simulink model "VCMGCM1962020b_v2"  (R2020b)
settings: Solver=FixedStepDiscrete  StartTime=0.0  StopTime=10.0  FixedStep=0.005  RelTol=1e-3  EnableMultiTasking=on
PreLoadFcn:
  | try, model_open; catch, disp('Error occurred while executing model pre-load callback: model_open.m'); disp('Please assure that the MATLAB working directory is set to the model directory before opening.'); end
InitFcn:
  | try, model_open; catch, end
undefined symbols (not defined in the file): Bridge, GCM, H, raptor_get_param_eval, raptor_get_safe_string, raptor_xcp_function
libraries: Blocks_lib x1165, Raptor_lib x665, simulink x62, VCM_lib x5
(part 4 of 23)

== system VCMGCM1962020b_v2/Fgnd/Control/Other/Cooling Pumps ==
  Data : Inport
  Bus Creator : BusCreator  Inputs=4
  Bus Selector1 : BusSelector  OutputSignals=Control.Mode.StartStop.ChgMode [Bool],Control.Mode.StartStop.RunMode [Bool]
  Bus Selector2 : BusSelector  OutputSignals=Control.Mode.StartStop.ChgMode [Bool],Control.Mode.StartStop.RunMode [Bool]
  Header : Blocks_lib/Header  width=Portrait  addtext=''
  Logical Operator : Logic  Inputs=3  AllPortsSameDT=off  OutDataTypeStr=boolean
  Logical Operator1 : Logic  Operator=OR  OutDataTypeStr=boolean
  Logical Operator2 : Logic  Inputs=3  AllPortsSameDT=off  OutDataTypeStr=boolean
  Logical Operator3 : Logic  Operator=OR  OutDataTypeStr=boolean
  Pump 1 Speed Request : Subsystem
  Pump 2 Speed Request : Subsystem
  raptor_adjustment : Raptor_lib/Data Storage/raptor_adjustment  paramName='CoolPump1EnblReqEnbl'  nameSource=Parameter  initValue=0  dataType=boolean  storage=Calibration  calDispType=Number  calEnum={'False', 'True'}  calGain=1  calOffset=0  calMax=inf  calMin=-inf  calFormat=''  calUnit='Bool'  calHelp='Cooling pump enable request enable'  calAccess=1  calFunction='Control | Cooling Loop'  calDispHeaders=off  calColHeaders={'Col1' 'Col2' 'Col3'}  calRowHeaders={'Row1' 'Row2' 'Row3'}
      settings: SourceProductName=Raptor
  raptor_adjustment1 : Raptor_lib/Data Storage/raptor_adjustment  paramName='CoolPump2EnblReqEnbl'  nameSource=Parameter  initValue=0  dataType=boolean  storage=Calibration  calDispType=Number  calEnum={'False', 'True'}  calGain=1  calOffset=0  calMax=inf  calMin=-inf  calFormat=''  calUnit='Bool'  calHelp='Cooling pump enable request enable'  calAccess=1  calFunction='Control | Cooling Loop'  calDispHeaders=off  calColHeaders={'Col1' 'Col2' 'Col3'}  calRowHeaders={'Row1' 'Row2' 'Row3'}
      settings: SourceProductName=Raptor
  Ctrl : Outport  VectorParamsAs1DForOutWhenUnconnected=off
  wires:
  Logical Operator1/1 -> Logical Operator/2
  Bus Selector1/1 -> Logical Operator1/1  "<ChgMode [Bool]>"
  Bus Selector1/2 -> Logical Operator1/2  "<RunMode [Bool]>"
  Bus Creator/1 -> Ctrl/1  "CoolPump"
  Pump 1 Speed Request/1(Bool) -> Logical Operator/3
  Logical Operator/1 -> Bus Creator/1  "CoolPump1EnblReq [Bool]"
  raptor_adjustment/1 -> Logical Operator/1
  Pump 1 Speed Request/2(%) -> Bus Creator/2  "CoolPump1SpdReq [%]"
  Pump 2 Speed Request/2(%) -> Bus Creator/4  "CoolPump2SpdReq [%]"
  raptor_adjustment1/1 -> Logical Operator2/1
  Pump 2 Speed Request/1(Bool) -> Logical Operator2/3
  Data/1 -> Bus Selector1/1, Pump 2 Speed Request/1(Data), Bus Selector2/1, Pump 1 Speed Request/1(Data)
  Bus Selector2/2 -> Logical Operator3/2  "<RunMode [Bool]>"
  Bus Selector2/1 -> Logical Operator3/1  "<ChgMode [Bool]>"
  Logical Operator3/1 -> Logical Operator2/2
  Logical Operator2/1 -> Bus Creator/3  "CoolPump2EnblReq [Bool]"

== system VCMGCM1962020b_v2/Fgnd/Control/Other/Heater ==
  Data : Inport
  Bus Creator : BusCreator  Inputs=3
  Bus Selector : BusSelector  OutputSignals=Control.Mode.StartStop.ChgMode [Bool],Control.Mode.StartStop.RunMode [Bool]
  Bus Selector1 : BusSelector  OutputSignals=VirtualSensors.Other.HeaterReq [Bool]
  Header : Blocks_lib/Header  width=Portrait  addtext=''
  Heater Pump : Stateflow chart  TreatAsAtomicUnit=on
  Logical Operator : Logic  Inputs=3  OutDataTypeStr=boolean
  Logical Operator1 : Logic  Operator=OR  OutDataTypeStr=boolean
  raptor_adjustment : Raptor_lib/Data Storage/raptor_adjustment  paramName='HeaterEnblReqEnbl'  nameSource=Parameter  initValue=0  dataType=boolean  storage=Calibration  calDispType=Number  calEnum={'False', 'True'}  calGain=1  calOffset=0  calMax=inf  calMin=-inf  calFormat=''  calUnit='Bool'  calHelp='Heater enable request enable'  calAccess=1  calFunction='Control | Heater'  calDispHeaders=off  calColHeaders={'Col1' 'Col2' 'Col3'}  calRowHeaders={'Row1' 'Row2' 'Row3'}
      settings: SourceProductName=Raptor
  raptor_adjustment1 : Raptor_lib/Data Storage/raptor_adjustment  paramName='HeaterOutletTempReq'  nameSource=Parameter  initValue=0  dataType=double  storage=Calibration  calDispType=Number  calEnum={'False', 'True'}  calGain=1.0  calOffset=0.0  calMax=inf  calMin=-inf  calFormat=''  calUnit='degC'  calHelp='Heater outlet temperature request'  calAccess=1  calFunction='Control | Heater'  calDispHeaders=off  calColHeaders={'Col1' 'Col2' 'Col3'}  calRowHeaders={'Row1' 'Row2' 'Row3'}
      settings: SourceProductName=Raptor
  raptor_adjustment2 : Raptor_lib/Data Storage/raptor_adjustment  paramName='HeaterPumpHoldTime'  nameSource=Parameter  initValue=0  dataType=uint16  storage=Calibration  calDispType=Number  calEnum={'Disabled', 'Enabled'}  calGain=samptime  calOffset=0  calMax=inf  calMin=-inf  calFormat='0.3'  calUnit='sec'  calHelp='Heater pump hold time (after heater turned off)'  calAccess=1  calFunction='Control | Heater'  calDispHeaders=off  calColHeaders={'Col1' 'Col2' 'Col3'}  calRowHeaders={'Row1' 'Row2' 'Row3'}
      settings: SourceProductName=Raptor
  raptor_adjustment3 : Raptor_lib/Data Storage/raptor_adjustment  paramName='HeaterPumpEnbl'  nameSource=Parameter  initValue=0  dataType=boolean  storage=Calibration  calDispType=Number  calEnum={'False', 'True'}  calGain=1  calOffset=0  calMax=inf  calMin=-inf  calFormat=''  calUnit='Bool'  calHelp='Heater pump enable'  calAccess=1  calFunction='Control | Heater'  calDispHeaders=off  calColHeaders={'Col1' 'Col2' 'Col3'}  calRowHeaders={'Row1' 'Row2' 'Row3'}
      settings: SourceProductName=Raptor
  Ctrl : Outport  VectorParamsAs1DForOutWhenUnconnected=off
  wires:
  Bus Selector1/1 -> Logical Operator/3  "<HeaterReq [Bool]>"
  Bus Creator/1 -> Ctrl/1  "Heater"
  Data/1 -> Bus Selector/1, Bus Selector1/1
  raptor_adjustment1/1 -> Bus Creator/2  "HeaterOutletTempReq [degC]"
  Bus Selector/2 -> Logical Operator1/2  "<RunMode [Bool]>"
  Bus Selector/1 -> Logical Operator1/1  "<ChgMode [Bool]>"
  Logical Operator1/1 -> Logical Operator/2
  raptor_adjustment/1 -> Logical Operator/1
  Heater Pump/1(Pump) -> Bus Creator/3  "HeaterPump [Bool]"
  raptor_adjustment2/1 -> Heater Pump/3(HoldTime)
  Logical Operator/1 -> Heater Pump/2(Heater), Bus Creator/1  "HeaterEnblReq [Bool]"
  raptor_adjustment3/1 -> Heater Pump/1(Enbl)

== system VCMGCM1962020b_v2/Fgnd/Control/Other/Other ==
  Data : Inport
  Bus Creator : BusCreator  Inputs=6
  Bus Selector : BusSelector  OutputSignals=Control.Mode.StartStop.OutptDiagEnbl [Bool]
  Bus Selector1 : BusSelector  OutputSignals=Control.Mode.StartStop.ModWake [Bool]
  Display : Subsystem
  FMWS : Subsystem
  Header : Blocks_lib/Header  width=Portrait  addtext=''
  Lights & Lamps : Subsystem
  Logical Operator : Logic  AllPortsSameDT=off  OutDataTypeStr=boolean
  Zero-Order Hold : ZeroOrderHold  SampleTime=-1
  raptor_adjustment : Raptor_lib/Data Storage/raptor_adjustment  paramName='HVILOutFrq_cal'  nameSource=Parameter  initValue=0  dataType=double  storage=Calibration  calDispType=Number  calEnum={'False', 'True'}  calGain=1.0  calOffset=0.0  calMax=inf  calMin=-inf  calFormat=''  calUnit='Hz'  calHelp='HVIL output frequency'  calAccess=1  calFunction='Control | Other'  calDispHeaders=off  calColHeaders={'Col1' 'Col2' 'Col3'}  calRowHeaders={'Row1' 'Row2' 'Row3'}
      settings: SourceProductName=Raptor
  raptor_adjustment1 : Raptor_lib/Data Storage/raptor_adjustment  paramName='SysWakeEnbl'  nameSource=Parameter  initValue=0  dataType=boolean  storage=Calibration  calDispType=Number  calEnum={'False', 'True'}  calGain=1  calOffset=0  calMax=inf  calMin=-inf  calFormat=''  calUnit='Bool'  calHelp='System wake enable'  calAccess=1  calFunction='Control | Other'  calDispHeaders=off  calColHeaders={'Col1' 'Col2' 'Col3'}  calRowHeaders={'Row1' 'Row2' 'Row3'}
      settings: SourceProductName=Raptor
  Ctrl : Outport  VectorParamsAs1DForOutWhenUnconnected=off
  wires:
  Bus Creator/1 -> Ctrl/1  "Other"
  Bus Selector/1 -> Zero-Order Hold/1  "<OutptDiagEnbl [Bool]>"
  Zero-Order Hold/1 -> Bus Creator/2  "MPDMWake [Bool]"
  raptor_adjustment/1 -> Bus Creator/1  "HVILOutFrq [Hz]"
  Lights & Lamps/1(Ctrl) -> Bus Creator/4
  Logical Operator/1 -> Bus Creator/3  "SysWake [Bool]"
  raptor_adjustment1/1 -> Logical Operator/1
  Data/1 -> Bus Selector1/1, FMWS/1(Data), Display/1(Data), Lights & Lamps/1(Data), Bus Selector/1
  Bus Selector1/1 -> Logical Operator/2  "<ModWake [Bool]>"
  Display/1(Ctrl) -> Bus Creator/5
  FMWS/1(Ctrl) -> Bus Creator/6

== system VCMGCM1962020b_v2/Fgnd/Control/Other/Park Pawl ==
  Data : Inport
  Bus Selector : BusSelector  OutputSignals=Control.Mode.PRNDMode [enum]
  CmprTo : Blocks_lib/CmprTo  op===  val='Prk'  enum=EnumLst.PRNDMode
  Header : Blocks_lib/Header  width=Portrait  addtext=''
  Logical Operator : Logic  OutDataTypeStr=boolean
  raptor_adjustment : Raptor_lib/Data Storage/raptor_adjustment  paramName='PrkPawlEnbl'  nameSource=Parameter  initValue=0  dataType=boolean  storage=Calibration  calDispType=Number  calEnum={'False', 'True'}  calGain=1  calOffset=0  calMax=inf  calMin=-inf  calFormat=''  calUnit='Bool'  calHelp='Park pawl enable'  calAccess=1  calFunction='Control | Park Pawl'  calDispHeaders=off  calColHeaders={'Col1' 'Col2' 'Col3'}  calRowHeaders={'Row1' 'Row2' 'Row3'}
      settings: SourceProductName=Raptor
  Bool : Outport  VectorParamsAs1DForOutWhenUnconnected=off
  wires:
  Data/1 -> Bus Selector/1
  Logical Operator/1 -> Bool/1
  Bus Selector/1 -> CmprTo/1  "<PRNDMode [enum]>"
  raptor_adjustment/1 -> Logical Operator/1
  CmprTo/1 -> Logical Operator/2

== system VCMGCM1962020b_v2/Fgnd/Control/Other/Power Steering Pump ==
  Data : Inport
  Bus Creator : BusCreator  Inputs=2
  Bus Selector : BusSelector  OutputSignals=Control.Mode.StartStop.RunMode [Bool],Control.Mode.PRNDMode [enum]
  Bus Selector1 : BusSelector  OutputSignals=VirtualSensors.Spd.VehSpd [kph]
  CmprTo : Blocks_lib/CmprTo  op=~=  val='Prk'  enum=EnumLst.PRNDMode
  Header : Blocks_lib/Header  width=Portrait  addtext=''
  Logical Operator : Logic  Inputs=3  OutDataTypeStr=boolean
  raptor_adjustment : Raptor_lib/Data Storage/raptor_adjustment  paramName='PSPInvtrEnblReqEnbl'  nameSource=Parameter  initValue=0  dataType=boolean  storage=Calibration  calDispType=Number  calEnum={'False', 'True'}  calGain=1  calOffset=0  calMax=inf  calMin=-inf  calFormat=''  calUnit='Bool'  calHelp='Power steering pump inverter enable request enable'  calAccess=1  calFunction='Control | Power Steering Pump'  calDispHeaders=off  calColHeaders={'Col1' 'Col2' 'Col3'}  calRowHeaders={'Row1' 'Row2' 'Row3'}
      settings: SourceProductName=Raptor
  raptor_table_1d : Raptor_lib/Table Lookup/raptor_table_1d  dataName='PSPMtrSpdReqTbl'  initValue=zeros(1,11)  dataType=double  storage=Calibration  initValueX=[1:11]  dataTypeXY=double  storageXY=Calibration  calVisible=on  showTable=on  calGain=1.0  calOffset=0.0  calMax=Inf  calMin=-Inf  calFormat='-1'  calUnit='rpm'  calHelp='Power steering pump motor speed request'  showBreakpoint=on  dataNameX='VehSpd11IdxArr'  calGainX=1.0  calOffsetX=0.0  calMaxX=Inf  calMinX=-Inf  calFormatX='-1'  calUnitX='kph'  calHelpX='Index array'  calAccess=1  calFunction='Control | Power Steering Pump'  measureEnable=on  mName='PSPMtrSpdReq'
      settings: SourceProductName=Raptor
  Ctrl : Outport  VectorParamsAs1DForOutWhenUnconnected=off
  wires:
  CmprTo/1 -> Logical Operator/3
  raptor_table_1d/1 -> Bus Creator/2  "PSPMtrSpdReq [rpm]"
  Logical Operator/1 -> Bus Creator/1  "PSPInvtrEnblReq [Bool]"
  Bus Creator/1 -> Ctrl/1  "PSPInvtr"
  Bus Selector1/1 -> raptor_table_1d/1  "<VehSpd [kph]>"
  Data/1 -> Bus Selector/1, Bus Selector1/1
  Bus Selector/1 -> Logical Operator/2  "<RunMode [Bool]>"
  Bus Selector/2 -> CmprTo/1  "<PRNDMode [enum]>"
  raptor_adjustment/1 -> Logical Operator/1

== system VCMGCM1962020b_v2/Fgnd/Control/PDU/High-Voltage Discharge Contactor ==
  Data : Inport
  Bus Selector : BusSelector  OutputSignals=Control.Mode.StartStop.HVDschg [Bool]
  HV Discharge : Stateflow chart  TreatAsAtomicUnit=on
  Header : Blocks_lib/Header  width=Portrait  addtext=''
  raptor_adjustment1 : Raptor_lib/Data Storage/raptor_adjustment  paramName='HVDschgMxTime'  nameSource=Parameter  initValue=0  dataType=uint16  storage=Calibration  calDispType=Number  calEnum={'Disabled', 'Enabled'}  calGain=samptime  calOffset=0  calMax=inf  calMin=-inf  calFormat='0.3'  calUnit='sec'  calHelp='High-voltage discharge maximum time (before setting fault)'  calAccess=1  calFunction='Control | PDU'  calDispHeaders=off  calColHeaders={'Col1' 'Col2' 'Col3'}  calRowHeaders={'Row1' 'Row2' 'Row3'}
      settings: SourceProductName=Raptor
  raptor_adjustment2 : Raptor_lib/Data Storage/raptor_adjustment  paramName='HVDschgRetryWaitTime'  nameSource=Parameter  initValue=0  dataType=uint16  storage=Calibration  calDispType=Number  calEnum={'Disabled', 'Enabled'}  calGain=samptime  calOffset=0  calMax=inf  calMin=-inf  calFormat='0.3'  calUnit='sec'  calHelp='High-voltage discharge retry wait time (after fault)'  calAccess=1  calFunction='Control | PDU'  calDispHeaders=off  calColHeaders={'Col1' 'Col2' 'Col3'}  calRowHeaders={'Row1' 'Row2' 'Row3'}
      settings: SourceProductName=Raptor
  Bool : Outport  VectorParamsAs1DForOutWhenUnconnected=off
  wires:
  Data/1 -> Bus Selector/1
  raptor_adjustment1/1 -> HV Discharge/2(MxTime)
  raptor_adjustment2/1 -> HV Discharge/3(RetryWaitTime)
  Bus Selector/1 -> HV Discharge/1(Enbl)  "<HVDschg [Bool]>"
  HV Discharge/1(Cntr) -> Bool/1

== system VCMGCM1962020b_v2/Fgnd/Control/PDU/Main  Contactor Cmd ==
  Data : Inport
  BusCreator : BusCreator  Inputs=2
  Enable : Subsystem
  HV Detect : Subsystem
  Header : Blocks_lib/Header  width=Portrait  addtext=''
  PreCharge Sequence : Stateflow chart  TreatAsAtomicUnit=on
  raptor_adjustment1 : Raptor_lib/Data Storage/raptor_adjustment  paramName=[nam 'PreChgMxTime']  nameSource=Parameter  initValue=0  dataType=uint16  storage=Calibration  calDispType=Number  calEnum={'Disabled', 'Enabled'}  calGain=samptime  calOffset=0  calMax=inf  calMin=-inf  calFormat='0.3'  calUnit='sec'  calHelp='Pre-charge maximum time (before setting fault)'  calAccess=1  calFunction=group  calDispHeaders=off  calColHeaders={'Col1' 'Col2' 'Col3'}  calRowHeaders={'Row1' 'Row2' 'Row3'}
      settings: SourceProductName=Raptor
  raptor_adjustment2 : Raptor_lib/Data Storage/raptor_adjustment  paramName=[nam 'PreChgRetryWaitTime']  nameSource=Parameter  initValue=0  dataType=uint16  storage=Calibration  calDispType=Number  calEnum={'Disabled', 'Enabled'}  calGain=samptime  calOffset=0  calMax=inf  calMin=-inf  calFormat='0.3'  calUnit='sec'  calHelp='Pre-charge retry wait time (after fault)'  calAccess=1  calFunction=group  calDispHeaders=off  calColHeaders={'Col1' 'Col2' 'Col3'}  calRowHeaders={'Row1' 'Row2' 'Row3'}
      settings: SourceProductName=Raptor
  raptor_adjustment3 : Raptor_lib/Data Storage/raptor_adjustment  paramName=[nam 'PreChgMxAttempts']  nameSource=Parameter  initValue=0  dataType=uint16  storage=Calibration  calDispType=Number  calEnum={'Disabled', 'Enabled'}  calGain=1  calOffset=0  calMax=inf  calMin=-inf  calFormat=''  calUnit='count'  calHelp='Pre-charge maximum attempts'  calAccess=1  calFunction=group  calDispHeaders=off  calColHeaders={'Col1' 'Col2' 'Col3'}  calRowHeaders={'Row1' 'Row2' 'Row3'}
      settings: SourceProductName=Raptor
  raptor_measurement : Raptor_lib/Data Storage/raptor_measurement  paramName=[nam 'MainCntrClosed']  nameSource=Parameter  calDispType=Number  calEnum={}  calGain=1.0  calOffset=0.0  calMax=inf  calMin=-inf  calFormat='-1'  calUnit='Bool'  calHelp='Main Cntr complete'  calAccess=1  calFunction=group  calVisible=on
      settings: SourceProductName=Raptor
  Ctrl : Outport  VectorParamsAs1DForOutWhenUnconnected=off
  wires:
  Data/1 -> Enable/1(Data), HV Detect/1(Data)
  raptor_adjustment3/1 -> PreCharge Sequence/5(MxAttempts)
  raptor_adjustment2/1 -> PreCharge Sequence/4(RetryWaitTime)
  raptor_adjustment1/1 -> PreCharge Sequence/3(MxTime)
  PreCharge Sequence/1(Complete) -> BusCreator/1, raptor_measurement/1  "MainPreChgComplete [Bool]"
  Enable/1(Bool) -> PreCharge Sequence/1(Enbl)  "MainPosCntr [Bool]"
  BusCreator/1 -> Ctrl/1  "MainCntrs"
  HV Detect/1(Full) -> PreCharge Sequence/2(HVDetect)
  PreCharge Sequence/2(CntrCmd) -> BusCreator/2  "MainPreChgCntr [Bool]"

== system VCMGCM1962020b_v2/Fgnd/Control/PDU/PDU Contactor Commands ==
  note: This Logic Determins if Contactors are commanded and confirmed
  Data : Inport
  BusCreator : BusCreator  Inputs=7
  CntrStatus : Subsystem
  Drive Inverter Contactor : Subsystem
  Enable : Subsystem
  HV Detect : Subsystem
  Header : Blocks_lib/Header  width=Portrait  addtext=''
  OR : Logic  Operator=OR  AllPortsSameDT=off  OutDataTypeStr=boolean
  Zero-Order Hold1 : ZeroOrderHold  SampleTime=-1
  Zero-Order Hold2 : ZeroOrderHold  SampleTime=-1
  Ctrl : Outport  VectorParamsAs1DForOutWhenUnconnected=off
  wires:
  Data/1 -> Drive Inverter Contactor/1(Data), Enable/1(Data), CntrStatus/1(Data), HV Detect/1(Data)
  Enable/1(RunEnbl) -> BusCreator/2, OR/1  "RunCntrs [Bool]"
  BusCreator/1 -> Ctrl/1  "PDUCntrs"
  Enable/2(ChrgEnbl) -> Zero-Order Hold2/1, OR/2  "ChrgCntr"
  Drive Inverter Contactor/1(Bool) -> BusCreator/1  "DrvInvtrCntrCmd [Bool]"
  Zero-Order Hold1/1 -> BusCreator/3  "DCDCCntrCmd [Bool]"
  OR/1 -> Zero-Order Hold1/1
  Zero-Order Hold2/1 -> BusCreator/4  "ChrgrCntrCmd [Bool]"
  HV Detect/1(Full) -> BusCreator/5  "HVDetected[Bool}"
  CntrStatus/1(RunClosed) -> BusCreator/6  "RunCntrsClosed [Bool]"
  CntrStatus/2(ChrgClosed) -> BusCreator/7  "ChrgCntrsClosed [Bool]"

== system VCMGCM1962020b_v2/Fgnd/Diagnostics/Diagnostics/A//C Compressor Fault ==
  Data : Inport
  Bus Selector : BusSelector  OutputSignals=Sensors.CAN.Other.ACC.ACCSTATUS1.ACCFltStat.ACCFltStatVld [Bool],VirtualSensors.PDU.MainCntrClosedVld [Bool]
  EvalDiag : Subsystem
  Header : Blocks_lib/Header  width=Portrait  addtext=''
  Logical Operator : Logic  AllPortsSameDT=off  OutDataTypeStr=boolean
  wires:
  Data/1 -> EvalDiag/1(Data), Bus Selector/1
  Bus Selector/1 -> Logical Operator/1  "<ACCFltStatVld [Bool]>"
  Bus Selector/2 -> Logical Operator/2  "<MainCntrClosedVld [Bool]>"
  Logical Operator/1 -> EvalDiag/Enable

== system VCMGCM1962020b_v2/Fgnd/Diagnostics/Diagnostics/Battery Cell Temperature (avg) High  ==
  Data : Inport
  Bus Selector : BusSelector  OutputSignals=VirtualSensors.Batt.BattCellTempAvgVld [Bool]
  EvalDiag : Subsystem
  Header : Blocks_lib/Header  width=Portrait  addtext=''
  wires:
  Bus Selector/1 -> EvalDiag/Enable  "<BattCellTempAvgVld [Bool]>"
  Data/1 -> Bus Selector/1, EvalDiag/1(Data)

== system VCMGCM1962020b_v2/Fgnd/Diagnostics/Diagnostics/Battery Cell Temperature (max) High ==
  Data : Inport
  Bus Selector : BusSelector  OutputSignals=VirtualSensors.Batt.BattCellTempMxVld [Bool]
  EvalDiag : Subsystem
  Header : Blocks_lib/Header  width=Portrait  addtext=''
  wires:
  Data/1 -> EvalDiag/1(Data), Bus Selector/1
  Bus Selector/1 -> EvalDiag/Enable  "<BattCellTempMxVld [Bool]>"

== system VCMGCM1962020b_v2/Fgnd/Diagnostics/Diagnostics/Battery Cell Voltage (max) High ==
  Data : Inport
  Bus Selector : BusSelector  OutputSignals=VirtualSensors.Batt.BattCellVoltMxVld [Bool]
  EvalDiag : Subsystem
  Header : Blocks_lib/Header  width=Portrait  addtext=''
  wires:
  Bus Selector/1 -> EvalDiag/Enable  "<BattCellVoltMxVld [Bool]>"
  Data/1 -> Bus Selector/1, EvalDiag/1(Data)

== system VCMGCM1962020b_v2/Fgnd/Diagnostics/Diagnostics/Battery Cell Voltage (min) Low ==
  Data : Inport
  Bus Selector : BusSelector  OutputSignals=VirtualSensors.Batt.BattCellVoltMnVld [Bool]
  EvalDiag : Subsystem
  Header : Blocks_lib/Header  width=Portrait  addtext=''
  wires:
  Data/1 -> EvalDiag/1(Data), Bus Selector/1
  Bus Selector/1 -> EvalDiag/Enable  "<BattCellVoltMnVld [Bool]>"

== system VCMGCM1962020b_v2/Fgnd/Diagnostics/Diagnostics/Battery Current High ==
  Data : Inport
  Bus Selector : BusSelector  OutputSignals=VirtualSensors.Batt.BattCurVld [Bool],VirtualSensors.Batt.BattDCLVld [Bool],VirtualSensors.Batt.BattCCLVld [Bool]
  EvalDiag : Subsystem
  Header : Blocks_lib/Header  width=Portrait  addtext=''
  Logical Operator : Logic  Inputs=3  AllPortsSameDT=off  OutDataTypeStr=boolean
  wires:
  Data/1 -> EvalDiag/1(Data), Bus Selector/1
  Bus Selector/3 -> Logical Operator/3  "<BattCCLVld [Bool]>"
  Bus Selector/1 -> Logical Operator/1  "<BattCurVld [Bool]>"
  Bus Selector/2 -> Logical Operator/2  "<BattDCLVld [Bool]>"
  Logical Operator/1 -> EvalDiag/Enable

== system VCMGCM1962020b_v2/Fgnd/Diagnostics/Diagnostics/Battery Fault ==
  Data : Inport
  Bus Selector : BusSelector  OutputSignals=VirtualSensors.Batt.BattFaultVld [Bool]
  EvalDiag : Subsystem
  Header : Blocks_lib/Header  width=Portrait  addtext=''
  wires:
  Data/1 -> Bus Selector/1, EvalDiag/1(Data)
  Bus Selector/1 -> EvalDiag/Enable  "<BattFaultVld [Bool]>"

== system VCMGCM1962020b_v2/Fgnd/Diagnostics/Diagnostics/CAN Bus Passive ==
  Data : Inport
  Bus Selector : BusSelector  OutputSignals=Control.Mode.StartStop.CANDiagEnbl [Bool]
  EvalDiag : Subsystem
  Header : Blocks_lib/Header  width=Portrait  addtext=''
  wires:
  Data/1 -> Bus Selector/1
  Bus Selector/1 -> EvalDiag/Enable  "<CANDiagEnbl [Bool]>"

== system VCMGCM1962020b_v2/Fgnd/Diagnostics/Diagnostics/Charger (off-board) Isolation Fault ==
  Data : Inport
  Bus Selector : BusSelector  OutputSignals=VirtualSensors.Chgr.OffBoard.OffBoardChgrIsoFaultVld [Bool]
  EvalDiag : Subsystem
  Header : Blocks_lib/Header  width=Portrait  addtext=''
  wires:
  Data/1 -> Bus Selector/1, EvalDiag/1(Data)
  Bus Selector/1 -> EvalDiag/Enable  "<OffBoardChgrIsoFaultVld [Bool]>"

== system VCMGCM1962020b_v2/Fgnd/Diagnostics/Diagnostics/Charger (on-board) Fault ==
  Data : Inport
  Bus Selector : BusSelector  OutputSignals=VirtualSensors.Chgr.OnBoard.OnBoardChgrFaultVld [Bool]
  EvalDiag : Subsystem
  Header : Blocks_lib/Header  width=Portrait  addtext=''
  wires:
  Data/1 -> Bus Selector/1, EvalDiag/1(Data)
  Bus Selector/1 -> EvalDiag/Enable  "<OnBoardChgrFaultVld [Bool]>"

== system VCMGCM1962020b_v2/Fgnd/Diagnostics/Diagnostics/Contactor SOH Faults ==
  Data : Inport
  Bus Selector : BusSelector  OutputSignals=VirtualSensors.PDU.MainPosCntrClosedVld [Bool],VirtualSensors.Batt.BattCurVld [Bool],VirtualSensors.PDU.MainPosCntrClosed [Bool],VirtualSensors.Batt.BattCur [A]
  Bus Selector1 : BusSelector  Commented=on  OutputSignals=VirtualSensors.PDU.MainNegCntrClosedVld [Bool],VirtualSensors.Batt.BattCurVld [Bool],VirtualSensors.PDU.MainNegCntrClosed [Bool],VirtualSensors.Batt.BattCur [A]
  Bus Selector2 : BusSelector  OutputSignals="VirtualSensors.PDU.DCDCCntrClosedVld  [Bool],VirtualSensors.Chgr.OffBoard.OffBoardChgrDCCurVld [Bool],VirtualSensors.PDU.DCDCCntrClosed [Bool],VirtualSensors.Chgr.OffBoard.OffBoardChgrDCCur [A]"
  Bus Selector3 : BusSelector  Commented=on  OutputSignals=VirtualSensors.PDU.DCChgNegCntrClosedVld [Bool],VirtualSensors.Chgr.OffBoard.OffBoardChgrDCCurVld [Bool],VirtualSensors.PDU.DCChgNegCntrClosed [Bool],VirtualSensors.Chgr.OffBoard.OffBoardChgrDCCur [A]
  Bus Selector4 : BusSelector  Commented=on  OutputSignals=VirtualSensors.PDU.DrvInvtrCntrClosedVld [Bool],VirtualSensors.DrvInvtr.DrvInvtrCurVld [Bool],VirtualSensors.PDU.DrvInvtrCntrClosed [Bool],VirtualSensors.DrvInvtr.DrvInvtrCur [A]
  CntrFltSOH : VCM_lib/CntrFltSOH  nam='MainPosCntr'  len=9  group='Diagnostics | System'  samptime=samptime
  CntrFltSOH1 : VCM_lib/CntrFltSOH  Commented=on  nam='MainNegCntr'  len=9  group='Diagnostics | System'  samptime=samptime
  CntrFltSOH2 : VCM_lib/CntrFltSOH  nam='DCChgPosCntr'  len=9  group='Diagnostics | System'  samptime=samptime
  CntrFltSOH3 : VCM_lib/CntrFltSOH  Commented=on  nam='DCChgNegCntr'  len=9  group='Diagnostics | System'  samptime=samptime
  CntrFltSOH4 : VCM_lib/CntrFltSOH  Commented=on  nam='DrvInvtrCntr'  len=9  group='Diagnostics | System'  samptime=samptime
  Header : Blocks_lib/Header  width=Portrait  addtext=''
  wires:
  Bus Selector4/4 -> CntrFltSOH4/4  "<DrvInvtrCur [A]>"
  Bus Selector4/3 -> CntrFltSOH4/3  "<DrvInvtrCntrClosed [Bool]>"
  Bus Selector4/2 -> CntrFltSOH4/2  "<DrvInvtrCurVld [Bool]>"
  Bus Selector4/1 -> CntrFltSOH4/1  "<DrvInvtrCntrClosedVld [Bool]>"
  Bus Selector3/4 -> CntrFltSOH3/4  "<OffBoardChgrDCCur [A]>"
  Bus Selector3/3 -> CntrFltSOH3/3  "<DCChgNegCntrClosed [Bool]>"
  Bus Selector3/2 -> CntrFltSOH3/2  "<OffBoardChgrDCCurVld [Bool]>"
  Bus Selector3/1 -> CntrFltSOH3/1  "<DCChgNegCntrClosedVld [Bool]>"
  Bus Selector2/4 -> CntrFltSOH2/4  "<OffBoardChgrDCCur [A]>"
  Bus Selector2/3 -> CntrFltSOH2/3  "<DCDCCntrClosed [Bool]>"
  Bus Selector2/2 -> CntrFltSOH2/2  "<OffBoardChgrDCCurVld [Bool]>"
  Bus Selector2/1 -> CntrFltSOH2/1  "<DCDCCntrClosedVld  [Bool]>"
  Bus Selector1/4 -> CntrFltSOH1/4  "<BattCur [A]>"
  Bus Selector1/3 -> CntrFltSOH1/3  "<MainNegCntrClosed [Bool]>"
  Bus Selector1/2 -> CntrFltSOH1/2  "<BattCurVld [Bool]>"
  Bus Selector1/1 -> CntrFltSOH1/1  "<MainNegCntrClosedVld [Bool]>"
  Bus Selector/4 -> CntrFltSOH/4  "<BattCur [A]>"
  Bus Selector/3 -> CntrFltSOH/3  "<MainPosCntrClosed [Bool]>"
  Bus Selector/2 -> CntrFltSOH/2  "<BattCurVld [Bool]>"
  Bus Selector/1 -> CntrFltSOH/1  "<MainPosCntrClosedVld [Bool]>"
  Data/1 -> Bus Selector/1, Bus Selector2/1, Bus Selector3/1, Bus Selector4/1, Bus Selector1/1

== system VCMGCM1962020b_v2/Fgnd/Diagnostics/Diagnostics/Contactor X-Checks ==
  Data : Inport
  AND : Logic  AllPortsSameDT=off  OutDataTypeStr=boolean
  Bus Selector : BusSelector  OutputSignals=Sensors.CAN.Batt.Status.StatusMsgVld [Bool]
  Bus Selector1 : BusSelector  OutputSignals=VirtualSensors.PDU.DrvInvtrCntrClosedVld [Bool],Control.PDU.PDUCntrs.RunCntrs [Bool]
  Bus Selector2 : BusSelector  OutputSignals="VirtualSensors.PDU.DCDCCntrClosedVld  [Bool]"
  Bus Selector3 : BusSelector  OutputSignals=VirtualSensors.PDU.ChrgrCntrClosedVld[Bool],Control.Mode.StartStop.ChgMode [Bool]
  Bus Selector4 : BusSelector  Commented=on  OutputSignals=VirtualSensors.PDU.DrvInvtrCntrClosedVld [Bool],Actuators.Actuators.PDU.DrvInvtrCntr.DrvInvtrCntrVld [Bool]
  Bus Selector5 : BusSelector  Commented=on  OutputSignals=VirtualSensors.PDU.HVDschgCntrClosedVld [Bool],Actuators.Actuators.PDU.HVDschgCntr.HVDschgCntrVld [Bool]
  EvalDiagChgrCntr : Subsystem
  EvalDiagDCDCCntr : Subsystem
  EvalDiagDrvInvtrCntr : Subsystem  Commented=on
  EvalDiagHVDschgCntr : Subsystem  Commented=on
  EvalDiagInvtrCntr : Subsystem
  EvalDiagMainCntr : Subsystem
  Header : Blocks_lib/Header  width=Portrait  addtext=''
  Logical Operator3 : Logic  AllPortsSameDT=off  OutDataTypeStr=boolean
  Logical Operator4 : Logic  Commented=on  AllPortsSameDT=off  OutDataTypeStr=boolean
  Logical Operator5 : Logic  Commented=on  AllPortsSameDT=off  OutDataTypeStr=boolean
  wires:
  Bus Selector5/1 -> Logical Operator5/1  "<HVDschgCntrClosedVld [Bool]>"
  Logical Operator5/1 -> EvalDiagHVDschgCntr/Enable
  Bus Selector5/2 -> Logical Operator5/2  "<HVDschgCntrVld [Bool]>"
  Logical Operator4/1 -> EvalDiagDrvInvtrCntr/Enable
  Bus Selector4/1 -> Logical Operator4/1  "<DrvInvtrCntrClosedVld [Bool]>"
  Bus Selector4/2 -> Logical Operator4/2  "<DrvInvtrCntrVld [Bool]>"
  Logical Operator3/1 -> EvalDiagChgrCntr/Enable
  Data/1 -> Bus Selector/1, EvalDiagInvtrCntr/1(Data), Bus Selector3/1, Bus Selector4/1, Bus Selector5/1, EvalDiagHVDschgCntr/1(Data), EvalDiagDrvInvtrCntr/1(Data), EvalDiagChgrCntr/1(Data), EvalDiagDCDCCntr/1(Data), Bus Selector2/1, Bus Selector1/1, EvalDiagMainCntr/1(Data)
  Bus Selector3/2 -> Logical Operator3/2  "<ChgMode [Bool]>"
  Bus Selector3/1 -> Logical Operator3/1  "<ChrgrCntrClosedVld[Bool]>"
  Bus Selector2/1 -> EvalDiagDCDCCntr/Enable  "<DCDCCntrClosedVld  [Bool]>"
  Bus Selector/1 -> EvalDiagMainCntr/Enable  "<StatusMsgVld [Bool]>"
  AND/1 -> EvalDiagInvtrCntr/Enable
  Bus Selector1/1 -> AND/1  "<DrvInvtrCntrClosedVld [Bool]>"
  Bus Selector1/2 -> AND/2  "<RunCntrs [Bool]>"

== system VCMGCM1962020b_v2/Fgnd/Diagnostics/Diagnostics/Cooling Pump Fault ==
  Data : Inport
  Bus Selector : BusSelector  Commented=on  OutputSignals=Sensors.CAN.Other.CoolPump1.CoolPump1DM1.CoolPump1DM1MsgVld [Bool]
  Bus Selector1 : BusSelector  Commented=on  OutputSignals=Sensors.CAN.Other.CoolPump2.CoolPump2DM1.CoolPump2DM1MsgVld [Bool]
  EvalDiag1 : Subsystem  Commented=on
  EvalDiag2 : Subsystem  Commented=on
  Header : Blocks_lib/Header  width=Portrait  addtext=''
  wires:
  Bus Selector/1 -> EvalDiag1/Enable  "<CoolPump1DM1MsgVld [Bool]>"
  Bus Selector1/1 -> EvalDiag2/Enable  "<CoolPump2DM1MsgVld [Bool]>"
  Data/1 -> Bus Selector/1, EvalDiag1/1(Data), Bus Selector1/1, EvalDiag2/1(Data)

== system VCMGCM1962020b_v2/Fgnd/Diagnostics/Diagnostics/DC//DC Converter Fault ==
  Data : Inport
  Bus Selector : BusSelector  OutputSignals=VirtualSensors.DCDC.DCDCFaultVld [Bool]
  EvalDiag : Subsystem
  Header : Blocks_lib/Header  width=Portrait  addtext=''
  wires:
  Data/1 -> Bus Selector/1, EvalDiag/1(Data)
  Bus Selector/1 -> EvalDiag/Enable  "<DCDCFaultVld [Bool]>"

== system VCMGCM1962020b_v2/Fgnd/Diagnostics/Diagnostics/DC//DC Converter X-Check ==
  Data : Inport
  Bus Selector : BusSelector  OutputSignals=Sensors.Sensors.Volt.DRVPVolt.DRVPVoltVld [Bool],Control.DCDC.DCDCEnblReq [Bool]
  EvalDiag : Subsystem
  Header : Blocks_lib/Header  width=Portrait  addtext=''
  Logical Operator : Logic  AllPortsSameDT=off  OutDataTypeStr=boolean
  wires:
  Bus Selector/1 -> Logical Operator/1  "<DRVPVoltVld [Bool]>"
  Bus Selector/2 -> Logical Operator/2  "<DCDCEnblReq [Bool]>"
  Data/1 -> Bus Selector/1, EvalDiag/1(Data)
  Logical Operator/1 -> EvalDiag/Enable

== system VCMGCM1962020b_v2/Fgnd/Diagnostics/Diagnostics/DRVP Voltage High//Low ==
  Data : Inport
  Bus Selector : BusSelector  OutputSignals=Sensors.Sensors.Volt.DRVPVolt.DRVPVoltVld [Bool],Control.Mode.StartStop.OutptDiagEnbl [Bool]
  EvalDiag : Subsystem
  Header : Blocks_lib/Header  width=Portrait  addtext=''
  Logical Operator : Logic  AllPortsSameDT=off  OutDataTypeStr=boolean
  wires:
  Bus Selector/2 -> Logical Operator/2  "<OutptDiagEnbl [Bool]>"
  Bus Selector/1 -> Logical Operator/1  "<DRVPVoltVld [Bool]>"
  Logical Operator/1 -> EvalDiag/Enable
  Data/1 -> Bus Selector/1, EvalDiag/1(Data)

== system VCMGCM1962020b_v2/Fgnd/Diagnostics/Diagnostics/Drive Inverter Fault ==
  Data : Inport
  Bus Selector : BusSelector  OutputSignals=VirtualSensors.DrvInvtr.DrvInvtrFaultVld [Bool]
  EvalDiag : Subsystem
  Header : Blocks_lib/Header  width=Portrait  addtext=''
  wires:
  Data/1 -> Bus Selector/1, EvalDiag/1(Data)
  Bus Selector/1 -> EvalDiag/Enable  "<DrvInvtrFaultVld [Bool]>"

== system VCMGCM1962020b_v2/Fgnd/Diagnostics/Diagnostics/Drive Motor Torque X-Check ==
  Data : Inport
  Bus Selector : BusSelector  OutputSignals=VirtualSensors.DrvInvtr.DrvMtrTrqVld [Bool],Control.DrvInvtr.DrvInvtrEnblReq [Bool]
  EvalDiag : Subsystem
  Header : Blocks_lib/Header  width=Portrait  addtext=''
  Logical Operator : Logic  AllPortsSameDT=off  OutDataTypeStr=boolean
  wires:
  Data/1 -> EvalDiag/1(Data), Bus Selector/1
  Bus Selector/2 -> Logical Operator/2  "<DrvInvtrEnblReq [Bool]>"
  Bus Selector/1 -> Logical Operator/1  "<DrvMtrTrqVld [Bool]>"
  Logical Operator/1 -> EvalDiag/Enable

== system VCMGCM1962020b_v2/Fgnd/Diagnostics/Diagnostics/E-Stop ==
  Data : Inport
  Bus Selector : BusSelector  OutputSignals=Sensors.Sensors.Driver.EStop1.EStop1Vld [Bool]
  Bus Selector1 : BusSelector  OutputSignals=Sensors.Sensors.Driver.EStop2.EStop2Vld [Bool]
  EvalDiag1 : Subsystem
  EvalDiag2 : Subsystem
  Header : Blocks_lib/Header  width=Portrait  addtext=''
  wires:
  Bus Selector/1 -> EvalDiag1/Enable  "<EStop1Vld [Bool]>"
  Data/1 -> Bus Selector1/1, EvalDiag2/1(Data), EvalDiag1/1(Data), Bus Selector/1
  Bus Selector1/1 -> EvalDiag2/Enable  "<EStop2Vld [Bool]>"

== system VCMGCM1962020b_v2/Fgnd/Diagnostics/Diagnostics/HV Bus Isolation Low ==
  Data : Inport
  Bus Selector : BusSelector  OutputSignals=VirtualSensors.PDU.HVBusIsoVld [Bool]
  EvalDiag : Subsystem
  Header : Blocks_lib/Header  width=Portrait  addtext=''
  wires:
  Data/1 -> Bus Selector/1, EvalDiag/1(Data)
  Bus Selector/1 -> EvalDiag/Enable  "<HVBusIsoVld [Bool]>"

== system VCMGCM1962020b_v2/Fgnd/Diagnostics/Diagnostics/HV Bus Voltage High ==
  Data : Inport
  Bus Selector : BusSelector  OutputSignals=VirtualSensors.PDU.HVBusVoltVld [Bool]
  EvalDiag : Subsystem
  Header : Blocks_lib/Header  width=Portrait  addtext=''
  wires:
  Data/1 -> Bus Selector/1, EvalDiag/1(Data)
  Bus Selector/1 -> EvalDiag/Enable  "<HVBusVoltVld [Bool]>"

== system VCMGCM1962020b_v2/Fgnd/Diagnostics/Diagnostics/HVIL X-Check ==
  Data : Inport
  Bus Selector : BusSelector  OutputSignals=Control.Mode.StartStop.InptDiagEnbl [Bool],Control.Mode.StartStop.OutptDiagEnbl [Bool]
  CntrSat : Blocks_lib/CntrSat  init=0  inc=1  typ=uint16  relop=>=  th_nam='HVILXChkWaitTime'  th_gain=samptime  th_units='sec'  th_help='Cross-check fault wait time (after output enabled)'  th_group='Diagnostics | System'
  EvalDiag : Subsystem
  Header : Blocks_lib/Header  width=Portrait  addtext=''
  Logical Operator : Logic  AllPortsSameDT=off  OutDataTypeStr=boolean
  Logical Operator1 : Logic  Operator=NOT  Inputs=1  OutDataTypeStr=boolean
  wires:
  Logical Operator/1 -> Logical Operator1/1, CntrSat/1
  Data/1 -> EvalDiag/1(Data), Bus Selector/1
  Bus Selector/2 -> Logical Operator/2  "<OutptDiagEnbl [Bool]>"
  Bus Selector/1 -> Logical Operator/1  "<InptDiagEnbl [Bool]>"
  Logical Operator1/1 -> CntrSat/2
  CntrSat/1 -> EvalDiag/Enable

== system VCMGCM1962020b_v2/Fgnd/Diagnostics/Diagnostics/Heater Fault ==
  Data : Inport
  Bus Selector : BusSelector  OutputSignals=Sensors.CAN.Other.Heater.HTR_OUT_1.HTR_STAT.HTR_STATVld [Bool],VirtualSensors.PDU.MainCntrClosedVld [Bool]
  EvalDiag : Subsystem
  Header : Blocks_lib/Header  width=Portrait  addtext=''
  Logical Operator : Logic  AllPortsSameDT=off  OutDataTypeStr=boolean
  wires:
  Data/1 -> Bus Selector/1, EvalDiag/1(Data)
  Bus Selector/1 -> Logical Operator/1  "<HTR_STATVld [Bool]>"
  Bus Selector/2 -> Logical Operator/2  "<MainCntrClosedVld [Bool]>"
  Logical Operator/1 -> EvalDiag/Enable

== system VCMGCM1962020b_v2/Fgnd/Diagnostics/Diagnostics/Inertia Switch ==
  Data : Inport
  Bus Selector : BusSelector  OutputSignals=Sensors.Sensors.Other.InertiaSw.InertiaSwVld [Bool]
  EvalDiag : Subsystem
  Header : Blocks_lib/Header  width=Portrait  addtext=''
  wires:
  Data/1 -> EvalDiag/1(Data), Bus Selector/1
  Bus Selector/1 -> EvalDiag/Enable  "<InertiaSwVld [Bool]>"

== system VCMGCM1962020b_v2/Fgnd/Diagnostics/Diagnostics/MPDM Fuse & Relay Faults ==
  note: Note: The 8-relay MPDM
      | configuration is as follows:
      |
      | Fuse #	Relay #	Connector/Pin #
      | 1		1		1D
      | 2		4		1C
      | 3		7		1F
      | 4		2		1B
      | 5		8		1H
      | 6		6		1G
      | 7		3		1E
      | 8		5		1A
      | 9		-		2D
      | 10		-		2C
      | 11		-		2G
      | 12		-		2H
      | 13		-		2E
      | 14		-		2F
      | 15		-		2B
      | 16		-		2A
      |
      | (Fuses 9-16 are for fused power only.)
  Data : Inport
  Bus Selector : BusSelector  OutputSignals=Sensors.CAN.Other.MPDM.MPDMFuseStatus.MPDMFuseStatusMsgVld [Bool]
  Bus Selector1 : BusSelector  OutputSignals=Sensors.CAN.Other.MPDM.MPDMRelayStatus.MPDMRelayStatusMsgVld [Bool]
  Header : Blocks_lib/Header  width=Portrait  addtext=''
  MPDM Fuse Faults : Subsystem
  MPDM Relay Faults : Subsystem
  wires:
  Data/1 -> MPDM Relay Faults/1(Data), Bus Selector1/1, MPDM Fuse Faults/1(Data), Bus Selector/1
  Bus Selector/1 -> MPDM Fuse Faults/Enable  "<MPDMFuseStatusMsgVld [Bool]>"
  Bus Selector1/1 -> MPDM Relay Faults/Enable  "<MPDMRelayStatusMsgVld [Bool]>"

== system VCMGCM1962020b_v2/Fgnd/Diagnostics/Diagnostics/MPRD Open//Short ==
  Data : Inport
  Bus Selector : BusSelector  OutputSignals=Control.Mode.StartStop.OutptDiagEnbl [Bool]
  EvalDiag : Subsystem
  Header : Blocks_lib/Header  width=Portrait  addtext=''
  wires:
  Data/1 -> Bus Selector/1
  Bus Selector/1 -> EvalDiag/Enable  "<OutptDiagEnbl [Bool]>"

== system VCMGCM1962020b_v2/Fgnd/Diagnostics/Diagnostics/Power Steering Pump Inverter Fault ==
  Data : Inport
  Bus Selector : BusSelector  OutputSignals=Sensors.CAN.Other.PSPInvtr.PSPInvtrHS2_Status_Feedback.PSPInvtrInverterStatus.PSPInvtrInverterStatusVld [Bool]
  EvalDiag : Subsystem
  Header : Blocks_lib/Header  width=Portrait  addtext=''
  wires:
  Data/1 -> Bus Selector/1, EvalDiag/1(Data)
  Bus Selector/1 -> EvalDiag/Enable  "<PSPInvtrInverterStatusVld [Bool]>"

== system VCMGCM1962020b_v2/Fgnd/Diagnostics/Diagnostics/XDRP Voltage High//Low ==
  Data : Inport
  Bus Selector : BusSelector  OutputSignals=Sensors.Sensors.Volt.XDRPVolt.XDRPVoltVld [Bool]
  EvalDiag : Subsystem
  Header : Blocks_lib/Header  width=Portrait  addtext=''
  wires:
  Data/1 -> Bus Selector/1, EvalDiag/1(Data)
  Bus Selector/1 -> EvalDiag/Enable  "<XDRPVoltVld [Bool]>"

== system VCMGCM1962020b_v2/Fgnd/Diagnostics/Fault Statuses/Clear All Faults ==
  Enable : EnablePort
  Constant : Constant  Value=boolean(0)
  Header : Blocks_lib/Header  width=Portrait  addtext=''
  raptor_data_write : Raptor_lib/Data Storage/raptor_data_write  dataName='ClearFaults'  dataShape=Scalar  idxSource=Input Port  idxRow=1  idxCol=1
      settings: SourceProductName=Raptor
  raptor_fault_clear : Raptor_lib/Faults/raptor_fault_clear  faultSource=All  faultName='myFault'
      settings: SourceProductName=Raptor
  wires:
  Constant/1 -> raptor_data_write/1

== system VCMGCM1962020b_v2/Fgnd/Diagnostics/Fault Statuses/Drive Cycle Logic ==
  note: Note: A drive cycle is considered complete when:
      | HVSysOff turns true due to VehPwrMode = Off (and it's not a ChgCycle), or
      | HVSysOff is already true and then VehPwrMode turns Off.
  Data : Inport
  Bus Selector : BusSelector  OutputSignals=Control.Mode.StartStop.HVSysOff [Bool],VirtualSensors.Driver.VehPwrMode [enum],Control.Mode.StartStop.ChgCycle [Bool]
  Bus Selector1 : BusSelector  OutputSignals=Control.Mode.StartStop.HVSysOff [Bool],VirtualSensors.Driver.VehPwrMode [enum]
  CmprTo : Blocks_lib/CmprTo  op===  val='Off'  enum=EnumLst.VehPwrMode
  CmprTo1 : Blocks_lib/CmprTo  op===  val='Off'  enum=EnumLst.VehPwrMode
  Detect Increase : simulink/Logic and Bit Operations/Detect Increase  vinit=0.0  OutDataTypeStr=boolean
  Detect Increase1 : simulink/Logic and Bit Operations/Detect Increase  vinit=0.0  OutDataTypeStr=boolean
  Drive Cycle Complete : Subsystem  TreatAsAtomicUnit=on
  Header : Blocks_lib/Header  width=Portrait  addtext=''
  Logical Operator : Logic  Operator=OR  AllPortsSameDT=off  OutDataTypeStr=boolean
  Logical Operator1 : Logic  Inputs=3  AllPortsSameDT=off  OutDataTypeStr=boolean
  Logical Operator2 : Logic  AllPortsSameDT=off  OutDataTypeStr=boolean
  Logical Operator3 : Logic  Operator=NOT  Inputs=3  AllPortsSameDT=off  OutDataTypeStr=boolean
  Unit Delay : UnitDelay  SampleTime=-1  HasFrameUpgradeWarning=on
  Warm-Up : Subsystem
  wires:
  Bus Selector/2 -> CmprTo/1  "<VehPwrMode [enum]>"
  Warm-Up/1(Bool) -> Drive Cycle Complete/1(WarmUp)
  Data/1 -> Warm-Up/1(Data), Bus Selector1/1, Bus Selector/1
  Bus Selector/1 -> Detect Increase/1  "<HVSysOff [Bool]>"
  Logical Operator1/1 -> Logical Operator/1
  Bus Selector1/2 -> CmprTo1/1  "<VehPwrMode [enum]>"
  Logical Operator2/1 -> Logical Operator/2
  CmprTo1/1 -> Detect Increase1/1
  Bus Selector1/1 -> Unit Delay/1  "<HVSysOff [Bool]>"
  Detect Increase1/1 -> Logical Operator2/2
  Unit Delay/1 -> Logical Operator2/1
  Logical Operator/1 -> Drive Cycle Complete/Enable
  Detect Increase/1 -> Logical Operator1/1
  CmprTo/1 -> Logical Operator1/2
  Bus Selector/3 -> Logical Operator3/1  "<ChgCycle [Bool]>"
  Logical Operator3/1 -> Logical Operator1/3

== system VCMGCM1962020b_v2/Fgnd/Diagnostics/Fault Statuses/Save NV ==
  Enable : EnablePort
  Constant : Constant  Value=boolean(0)
  Function-Call Generator : simulink/Ports & Subsystems/Function-Call Generator  sample_time=-1  numberOfIterations=1  DisallowWideOutput=off
  Header : Blocks_lib/Header  width=Portrait  addtext=''
  raptor_data_write : Raptor_lib/Data Storage/raptor_data_write  dataName='SaveNV'  dataShape=Scalar  idxSource=Input Port  idxRow=1  idxCol=1
      settings: SourceProductName=Raptor
  raptor_store_nv : Raptor_lib/Data Storage/raptor_store_nv  null=0
      settings: SourceProductName=Raptor
  wires:
  Function-Call Generator/1 -> raptor_store_nv/Trigger
  Constant/1 -> raptor_data_write/1
